simulink model "car_simulink"  (R2016a)
settings: Solver=FixedStepAuto  StartTime=0.0  StopTime=inf  RelTol=1e-3
libraries: arduinolib x8
settings Model: SimulationMode=external  ExtModeTrigDuration=2  Creator=Ahmed Refaat  LastModifiedBy=Ahmed Refaat
settings OptimizationCC: OptimizeModelRefInitCode=on  LifeSpan=Inf  MaxStackSize=64
settings HardwareCC: ProdBitPerInt=16  ProdBitPerPointer=16  ProdLargestAtomicFloat=None  ProdWordSize=8  ProdHWDeviceType=Atmel->AVR
settings RTWCC: SystemTargetFile=ert.tlc  HardwareBoard=Arduino Uno  TemplateMakefile=ert_default_tmf  GenerateReport=on  Toolchain=Arduino AVR v1.6.1  BuildConfiguration=Faster Runs  IncludeHyperlinkInReport=on  LaunchReport=on  GenerateTraceInfo=on  GenerateTraceReport=on  GenerateTraceReportSl=on  GenerateTraceReportSf=on  GenerateTraceReportEml=on
settings CodeAppCC: ForceParamTrailComments=on  IgnoreCustomStorageClasses=off  OperatorAnnotations=on  SimulinkDataObjDesc=on  SFDataObjDesc=on  MATLABFcnDesc=on  InsertBlockDesc=on  MATLABSourceComments=on
settings ERTTargetCC: SupportContinuousTime=on  SupportVariableSizeSignals=on

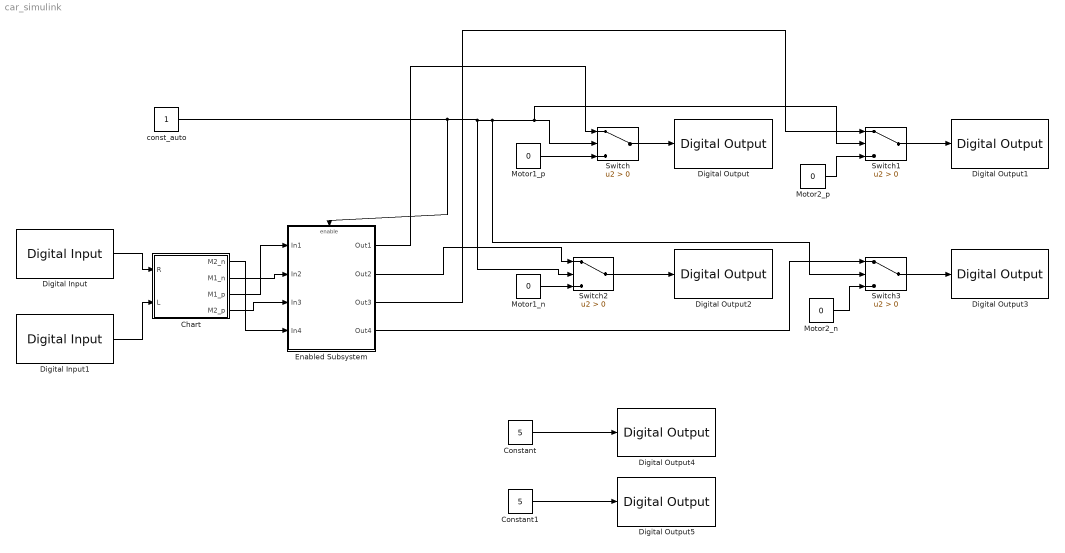
== system car_simulink ==
  Chart : Stateflow chart  TreatAsAtomicUnit=on
  Constant : Constant  Value=5
  Constant1 : Constant  Value=5
  Digital Input : arduinolib/Digital Input  pinNumber=7  sampleTime=1  blockPlatform=arduino
  Digital Input1 : arduinolib/Digital Input  pinNumber=8  sampleTime=1  blockPlatform=arduino
  Digital Output : arduinolib/Digital Output  pinNumber=2  blockPlatform=arduino
  Digital Output1 : arduinolib/Digital Output  pinNumber=4  blockPlatform=arduino
  Digital Output2 : arduinolib/Digital Output  pinNumber=3  blockPlatform=arduino
  Digital Output3 : arduinolib/Digital Output  pinNumber=5  blockPlatform=arduino
  Digital Output4 : arduinolib/Digital Output  pinNumber=9  blockPlatform=arduino
  Digital Output5 : arduinolib/Digital Output  pinNumber=10  blockPlatform=arduino
  Enabled Subsystem : Subsystem  TreatAsAtomicUnit=on
  Motor1_n : Constant  Value=0
  Motor1_p : Constant  Value=0
  Motor2_n : Constant  Value=0
  Motor2_p : Constant  Value=0
  Switch{,1..3} (4 alike) : Switch  Criteria=u2 > Threshold
  const_auto : Constant
  wires:
  Constant/1 -> Digital Output4/1
  Constant1/1 -> Digital Output5/1
  const_auto/1 -> Enabled Subsystem/Enable, Switch2/2, Switch3/2, Switch1/2, Switch/2
  Motor1_p/1 -> Switch/3
  Switch/1 -> Digital Output/1
  Switch1/1 -> Digital Output1/1
  Motor2_p/1 -> Switch1/3
  Switch2/1 -> Digital Output2/1
  Motor1_n/1 -> Switch2/3
  Motor2_n/1 -> Switch3/3
  Switch3/1 -> Digital Output3/1
  Enabled Subsystem/1(Out1) -> Switch/1
  Enabled Subsystem/2(Out2) -> Switch2/1
  Enabled Subsystem/3(Out3) -> Switch1/1
  Enabled Subsystem/4(Out4) -> Switch3/1
  Digital Input/1 -> Chart/1(R)
  Digital Input1/1 -> Chart/2(L)
  Chart/3(M1_p) -> Enabled Subsystem/1(In1)
  Chart/2(M1_n) -> Enabled Subsystem/2(In2)
  Chart/4(M2_p) -> Enabled Subsystem/3(In3)
  Chart/1(M2_n) -> Enabled Subsystem/4(In4)

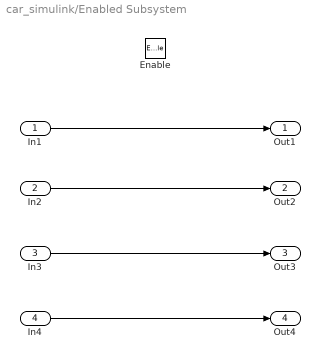
== system car_simulink/Enabled Subsystem ==
  In1 : Inport
  In2 : Inport  Port=2
  In3 : Inport  Port=3
  In4 : Inport  Port=4
  Enable : EnablePort
  Out1 : Outport
  Out2 : Outport  Port=2
  Out3 : Outport  Port=3
  Out4 : Outport  Port=4
  wires:
  In1/1 -> Out1/1
  In2/1 -> Out2/1
  In3/1 -> Out3/1
  In4/1 -> Out4/1

== stateflow chart car_simulink/Chart ==
  state Forward
    entry: M1_p =1
    M1_n =0
    M2_p =1
    M2_n =0
  state Left
    entry: M1_p =0
    M1_n =0
    M2_p =1
    M2_n =0
  state Right
    entry:  M1_p =1
    M1_n =0
    M2_p =0
    M2_n =0
  state Stop
    entry:  M1_p =0
    M1_n =0
    M2_p =0
    M2_n =0
  (default) -> Forward
  Forward -> Right [order 1] : [L==1 && R==0]
  Left -> Forward [order 1] : [L==1 && R==1]
  Forward -> Left [order 3] : [L==0 && R==1]
  Stop -> Forward [order 2] : [L==1 && R==1]
  Forward -> Stop [order 2] : [L==0 && R==0]
  Right -> Forward [order 3] : [L==1 && R==1]
  Right -> Left [order 1] : [L==0 && R==1]
  Left -> Right [order 2] : [L==1 && R==0]
  Left -> Stop [order 3] : [L==0 && R==0]
  Stop -> Left [order 1] : [L==0 && R==1]
  Stop -> Right [order 3] : [L==1 && R==0]
  Right -> Stop [order 2] : [L==0 && R==0]
  data: M2_n output; M1_n output; M1_p output; M2_p output; R input; L input
